simulink model "car"  (R2021a)
settings: Solver=VariableStepAuto  StartTime=0.0  StopTime=10.0  RelTol=1e-3
settings Model: Creator=smrh1  LastModifiedBy=smrh1

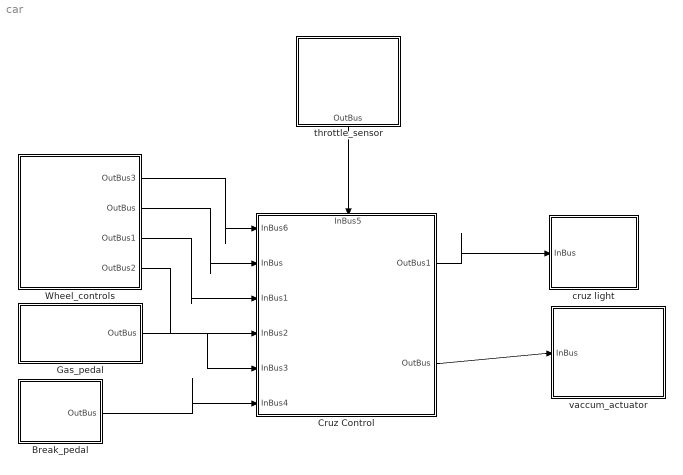
== system car ==
  Break_pedal : Subsystem
      settings: PortSchema="{\"entries\":[{\"content\":{\"headerSize\":26,\"margin\":15,\"minimumSpacing\":25,\"sides\":[{\"content\":{\"connectorIds\":[]},\"type\":\"ConnectorPlacement.EquallySpacedRectSide\",\"uuid\":\"6472313b-455b-4d2f-9eaa-19f0e43a9d41\"},{\"content\":{\"connectorIds\":[\"Out1\"],\"side\":\"RIGHT\"},\"type\":\"ConnectorPlacement.EquallySpacedRectSide\",\"uuid\":\"0bb4b84f-a849-43c7-b807-c30cbc689ce2\"},{\"content\":{\"connectorIds\":[],\"side\":\"TOP\"},\"type\":\"ConnectorPlacement.EquallySpacedRectSide\",\"uuid\":\"136300d7-46ce-438e-aee5-bc57502263b3\"}]},\"type\":\"ConnectorPlacement.EquallySpacedConnector\",\"uuid\":\"08cdd62d-e07b-40ae-9685-722663ceea2d\"}],\"packageUris\":[\"http://schema.mathworks.com/mf0/Connector/R2020b\"],\"version\":\"1.0\"}"
  Cruz Control : Subsystem
      settings: PortSchema="{\"entries\":[{\"content\":{\"headerSize\":26,\"margin\":15,\"minimumSpacing\":25,\"sides\":[{\"content\":{\"connectorIds\":[\"In1\",\"In5\",\"In3\",\"In4\",\"In6\",\"In7\"]},\"type\":\"ConnectorPlacement.EquallySpacedRectSide\",\"uuid\":\"6472313b-455b-4d2f-9eaa-19f0e43a9d41\"},{\"content\":{\"connectorIds\":[\"Out1\",\"Out2\"],\"side\":\"RIGHT\"},\"type\":\"ConnectorPlacement.EquallySpacedRectSide\",\"uuid\":\"0bb4b84f-a849-43c7-b807-c30cbc689ce2\"},{\"content\":{\"connectorIds\":[\"In2\"],\"side\":\"TOP\"},\"type\":\"ConnectorPlacement.EquallySpacedRectSide\",\"uuid\":\"136300d7-46ce-438e-aee5-bc57502263b3\"},{\"content\":{\"connectorIds\":[],\"side\":\"BOTTOM\"},\"type\":\"ConnectorPlacement.EquallySpacedRectSide\",\"uuid\":\"9109190a-ab23-468c-b16c-34fb84e28b1e\"}]},\"type\":\"ConnectorPlacement.EquallySpacedConnector\",\"uuid\":\"08cdd62d-e07b-40ae-9685-722663ceea2d\"}],\"packageUris\":[\"http://schema.mathworks.com/mf0/Connector/R2020b\"],\"version\":\"1.0\"}"
  Gas_pedal : Subsystem
      settings: PortSchema="{\"entries\":[{\"content\":{\"headerSize\":26,\"margin\":15,\"minimumSpacing\":25,\"sides\":[{\"content\":{\"connectorIds\":[]},\"type\":\"ConnectorPlacement.EquallySpacedRectSide\",\"uuid\":\"6472313b-455b-4d2f-9eaa-19f0e43a9d41\"},{\"content\":{\"connectorIds\":[\"Out1\"],\"side\":\"RIGHT\"},\"type\":\"ConnectorPlacement.EquallySpacedRectSide\",\"uuid\":\"0bb4b84f-a849-43c7-b807-c30cbc689ce2\"},{\"content\":{\"connectorIds\":[],\"side\":\"TOP\"},\"type\":\"ConnectorPlacement.EquallySpacedRectSide\",\"uuid\":\"136300d7-46ce-438e-aee5-bc57502263b3\"}]},\"type\":\"ConnectorPlacement.EquallySpacedConnector\",\"uuid\":\"08cdd62d-e07b-40ae-9685-722663ceea2d\"}],\"packageUris\":[\"http://schema.mathworks.com/mf0/Connector/R2020b\"],\"version\":\"1.0\"}"
  Wheel_controls : Subsystem
      settings: PortSchema="{\"entries\":[{\"content\":{\"headerSize\":26,\"margin\":15,\"minimumSpacing\":25,\"sides\":[{\"content\":{\"connectorIds\":[]},\"type\":\"ConnectorPlacement.EquallySpacedRectSide\",\"uuid\":\"af031d74-65d2-4252-81e5-6d9a1fd8149f\"},{\"content\":{\"connectorIds\":[\"Out1\",\"Out2\",\"Out3\",\"Out4\"],\"side\":\"RIGHT\"},\"type\":\"ConnectorPlacement.EquallySpacedRectSide\",\"uuid\":\"daede40a-d3c3-4ef5-9610-a569ab521095\"},{\"content\":{\"connectorIds\":[],\"side\":\"TOP\"},\"type\":\"ConnectorPlacement.EquallySpacedRectSide\",\"uuid\":\"d81e0d84-460b-4569-b916-0cc5afe47905\"}]},\"type\":\"ConnectorPlacement.EquallySpacedConnector\",\"uuid\":\"ddc853b2-7e74-44f1-90da-04896d4738c6\"}],\"packageUris\":[\"http://schema.mathworks.com/mf0/Connector/R2020b\"],\"version\":\"1.0\"}"
  cruz light : Subsystem
      settings: PortSchema="{\"entries\":[{\"content\":{\"headerSize\":26,\"margin\":15,\"minimumSpacing\":25,\"sides\":[{\"content\":{\"connectorIds\":[\"In1\"]},\"type\":\"ConnectorPlacement.EquallySpacedRectSide\",\"uuid\":\"6472313b-455b-4d2f-9eaa-19f0e43a9d41\"},{\"content\":{\"connectorIds\":[],\"side\":\"RIGHT\"},\"type\":\"ConnectorPlacement.EquallySpacedRectSide\",\"uuid\":\"0bb4b84f-a849-43c7-b807-c30cbc689ce2\"},{\"content\":{\"connectorIds\":[],\"side\":\"TOP\"},\"type\":\"ConnectorPlacement.EquallySpacedRectSide\",\"uuid\":\"136300d7-46ce-438e-aee5-bc57502263b3\"}]},\"type\":\"ConnectorPlacement.EquallySpacedConnector\",\"uuid\":\"08cdd62d-e07b-40ae-9685-722663ceea2d\"}],\"packageUris\":[\"http://schema.mathworks.com/mf0/Connector/R2020b\"],\"version\":\"1.0\"}"
  throttle_sensor : Subsystem
      settings: PortSchema="{\"entries\":[{\"content\":{\"headerSize\":26,\"margin\":15,\"minimumSpacing\":25,\"sides\":[{\"content\":{\"connectorIds\":[]},\"type\":\"ConnectorPlacement.EquallySpacedRectSide\",\"uuid\":\"6472313b-455b-4d2f-9eaa-19f0e43a9d41\"},{\"content\":{\"connectorIds\":[],\"side\":\"RIGHT\"},\"type\":\"ConnectorPlacement.EquallySpacedRectSide\",\"uuid\":\"0bb4b84f-a849-43c7-b807-c30cbc689ce2\"},{\"content\":{\"connectorIds\":[],\"side\":\"TOP\"},\"type\":\"ConnectorPlacement.EquallySpacedRectSide\",\"uuid\":\"136300d7-46ce-438e-aee5-bc57502263b3\"},{\"content\":{\"connectorIds\":[\"Out1\"],\"side\":\"BOTTOM\"},\"type\":\"ConnectorPlacement.EquallySpacedRectSide\",\"uuid\":\"8eadb317-004d-496f-aa52-9a68b828bcdc\"}]},\"type\":\"ConnectorPlacement.EquallySpacedConnector\",\"uuid\":\"08cdd62d-e07b-40ae-9685-722663ceea2d\"}],\"packageUris\":[\"http://schema.mathworks.com/mf0/Connector/R2020b\"],\"version\":\"1.0\"}"
  vaccum_actuator : Subsystem
      settings: PortSchema="{\"entries\":[{\"content\":{\"headerSize\":26,\"margin\":15,\"minimumSpacing\":25,\"sides\":[{\"content\":{\"connectorIds\":[\"In1\"]},\"type\":\"ConnectorPlacement.EquallySpacedRectSide\",\"uuid\":\"6472313b-455b-4d2f-9eaa-19f0e43a9d41\"},{\"content\":{\"connectorIds\":[],\"side\":\"RIGHT\"},\"type\":\"ConnectorPlacement.EquallySpacedRectSide\",\"uuid\":\"0bb4b84f-a849-43c7-b807-c30cbc689ce2\"},{\"content\":{\"connectorIds\":[],\"side\":\"TOP\"},\"type\":\"ConnectorPlacement.EquallySpacedRectSide\",\"uuid\":\"136300d7-46ce-438e-aee5-bc57502263b3\"}]},\"type\":\"ConnectorPlacement.EquallySpacedConnector\",\"uuid\":\"08cdd62d-e07b-40ae-9685-722663ceea2d\"}],\"packageUris\":[\"http://schema.mathworks.com/mf0/Connector/R2020b\"],\"version\":\"1.0\"}"
  wires:
  Gas_pedal/1(OutBus) -> Cruz Control/6(InBus3)
  Cruz Control/1(OutBus1) -> cruz light/1(InBus)
  Break_pedal/1(OutBus) -> Cruz Control/7(InBus4)
  Cruz Control/2(OutBus) -> vaccum_actuator/1(InBus)
  throttle_sensor/1(OutBus) -> Cruz Control/2(InBus5)
  Wheel_controls/2(OutBus) -> Cruz Control/5(InBus)
  Wheel_controls/3(OutBus1) -> Cruz Control/3(InBus1)
  Wheel_controls/4(OutBus2) -> Cruz Control/4(InBus2)
  Wheel_controls/1(OutBus3) -> Cruz Control/1(InBus6)

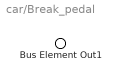
== system car/Break_pedal ==
  Bus Element Out1 : Outport  PortName=OutBus

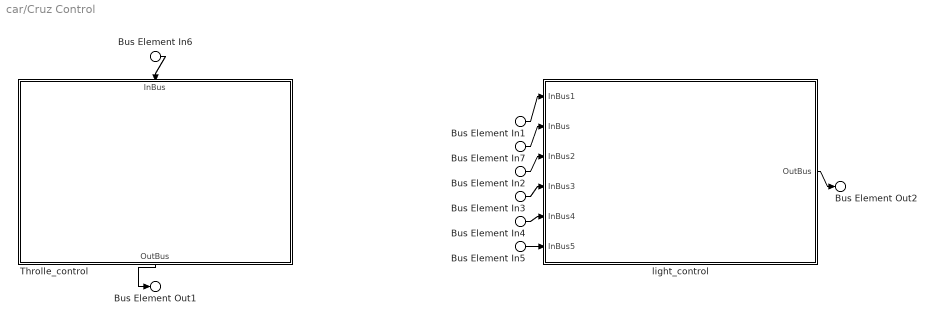
== system car/Cruz Control ==
  Bus Element In7 : Inport  PortName=InBus6
  Bus Element In6 : Inport  Port=2  PortName=InBus5
  Bus Element In2 : Inport  Port=3  PortName=InBus1
  Bus Element In3 : Inport  Port=4  PortName=InBus2
  Bus Element In1 : Inport  Port=5  PortName=InBus
  Bus Element In4 : Inport  Port=6  PortName=InBus3
  Bus Element In5 : Inport  Port=7  PortName=InBus4
  Throlle_control : Subsystem
      settings: PortSchema="{\"entries\":[{\"content\":{\"headerSize\":26,\"margin\":15,\"minimumSpacing\":25,\"sides\":[{\"content\":{\"connectorIds\":[]},\"type\":\"ConnectorPlacement.EquallySpacedRectSide\",\"uuid\":\"6472313b-455b-4d2f-9eaa-19f0e43a9d41\"},{\"content\":{\"connectorIds\":[],\"side\":\"RIGHT\"},\"type\":\"ConnectorPlacement.EquallySpacedRectSide\",\"uuid\":\"0bb4b84f-a849-43c7-b807-c30cbc689ce2\"},{\"content\":{\"connectorIds\":[\"In1\"],\"side\":\"TOP\"},\"type\":\"ConnectorPlacement.EquallySpacedRectSide\",\"uuid\":\"136300d7-46ce-438e-aee5-bc57502263b3\"},{\"content\":{\"connectorIds\":[\"Out1\"],\"side\":\"BOTTOM\"},\"type\":\"ConnectorPlacement.EquallySpacedRectSide\",\"uuid\":\"47a51370-8899-40a2-9cda-cea4c92ab7c8\"}]},\"type\":\"ConnectorPlacement.EquallySpacedConnector\",\"uuid\":\"08cdd62d-e07b-40ae-9685-722663ceea2d\"}],\"packageUris\":[\"http://schema.mathworks.com/mf0/Connector/R2020b\"],\"version\":\"1.0\"}"
  light_control : Subsystem
      settings: PortSchema="{\"entries\":[{\"content\":{\"headerSize\":26,\"margin\":15,\"minimumSpacing\":25,\"sides\":[{\"content\":{\"connectorIds\":[\"In1\",\"In2\",\"In3\",\"In4\",\"In5\",\"In6\"]},\"type\":\"ConnectorPlacement.EquallySpacedRectSide\",\"uuid\":\"6472313b-455b-4d2f-9eaa-19f0e43a9d41\"},{\"content\":{\"connectorIds\":[\"Out1\"],\"side\":\"RIGHT\"},\"type\":\"ConnectorPlacement.EquallySpacedRectSide\",\"uuid\":\"0bb4b84f-a849-43c7-b807-c30cbc689ce2\"},{\"content\":{\"connectorIds\":[],\"side\":\"TOP\"},\"type\":\"ConnectorPlacement.EquallySpacedRectSide\",\"uuid\":\"136300d7-46ce-438e-aee5-bc57502263b3\"}]},\"type\":\"ConnectorPlacement.EquallySpacedConnector\",\"uuid\":\"08cdd62d-e07b-40ae-9685-722663ceea2d\"}],\"packageUris\":[\"http://schema.mathworks.com/mf0/Connector/R2020b\"],\"version\":\"1.0\"}"
  Bus Element Out2 : Outport  PortName=OutBus1
  Bus Element Out1 : Outport  Port=2  PortName=OutBus
  wires:
  Bus Element In7/1 -> light_control/2(InBus)
  Bus Element In1/1 -> light_control/1(InBus1)
  Bus Element In2/1 -> light_control/3(InBus2)
  Bus Element In3/1 -> light_control/4(InBus3)
  Bus Element In4/1 -> light_control/5(InBus4)
  Bus Element In5/1 -> light_control/6(InBus5)
  light_control/1(OutBus) -> Bus Element Out2/1
  Bus Element In6/1 -> Throlle_control/1(InBus)
  Throlle_control/1(OutBus) -> Bus Element Out1/1

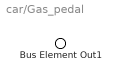
== system car/Gas_pedal ==
  Bus Element Out1 : Outport  PortName=OutBus

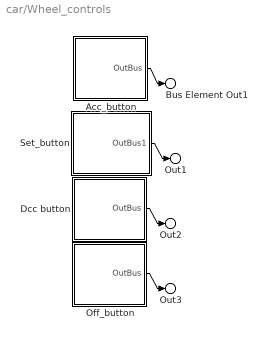
== system car/Wheel_controls ==
  Acc_button : Subsystem
      settings: PortSchema="{\"entries\":[{\"content\":{\"headerSize\":26,\"margin\":15,\"minimumSpacing\":25,\"sides\":[{\"content\":{\"connectorIds\":[]},\"type\":\"ConnectorPlacement.EquallySpacedRectSide\",\"uuid\":\"6472313b-455b-4d2f-9eaa-19f0e43a9d41\"},{\"content\":{\"connectorIds\":[\"Out1\"],\"side\":\"RIGHT\"},\"type\":\"ConnectorPlacement.EquallySpacedRectSide\",\"uuid\":\"0bb4b84f-a849-43c7-b807-c30cbc689ce2\"},{\"content\":{\"connectorIds\":[],\"side\":\"TOP\"},\"type\":\"ConnectorPlacement.EquallySpacedRectSide\",\"uuid\":\"136300d7-46ce-438e-aee5-bc57502263b3\"}]},\"type\":\"ConnectorPlacement.EquallySpacedConnector\",\"uuid\":\"08cdd62d-e07b-40ae-9685-722663ceea2d\"}],\"packageUris\":[\"http://schema.mathworks.com/mf0/Connector/R2020b\"],\"version\":\"1.0\"}"
  Dcc button : Subsystem
      settings: PortSchema="{\"entries\":[{\"content\":{\"headerSize\":26,\"margin\":15,\"minimumSpacing\":25,\"sides\":[{\"content\":{\"connectorIds\":[]},\"type\":\"ConnectorPlacement.EquallySpacedRectSide\",\"uuid\":\"6472313b-455b-4d2f-9eaa-19f0e43a9d41\"},{\"content\":{\"connectorIds\":[\"Out1\"],\"side\":\"RIGHT\"},\"type\":\"ConnectorPlacement.EquallySpacedRectSide\",\"uuid\":\"0bb4b84f-a849-43c7-b807-c30cbc689ce2\"},{\"content\":{\"connectorIds\":[],\"side\":\"TOP\"},\"type\":\"ConnectorPlacement.EquallySpacedRectSide\",\"uuid\":\"136300d7-46ce-438e-aee5-bc57502263b3\"}]},\"type\":\"ConnectorPlacement.EquallySpacedConnector\",\"uuid\":\"08cdd62d-e07b-40ae-9685-722663ceea2d\"}],\"packageUris\":[\"http://schema.mathworks.com/mf0/Connector/R2020b\"],\"version\":\"1.0\"}"
  Off_button : Subsystem
      settings: PortSchema="{\"entries\":[{\"content\":{\"headerSize\":26,\"margin\":15,\"minimumSpacing\":25,\"sides\":[{\"content\":{\"connectorIds\":[]},\"type\":\"ConnectorPlacement.EquallySpacedRectSide\",\"uuid\":\"6472313b-455b-4d2f-9eaa-19f0e43a9d41\"},{\"content\":{\"connectorIds\":[\"Out1\"],\"side\":\"RIGHT\"},\"type\":\"ConnectorPlacement.EquallySpacedRectSide\",\"uuid\":\"0bb4b84f-a849-43c7-b807-c30cbc689ce2\"},{\"content\":{\"connectorIds\":[],\"side\":\"TOP\"},\"type\":\"ConnectorPlacement.EquallySpacedRectSide\",\"uuid\":\"136300d7-46ce-438e-aee5-bc57502263b3\"}]},\"type\":\"ConnectorPlacement.EquallySpacedConnector\",\"uuid\":\"08cdd62d-e07b-40ae-9685-722663ceea2d\"}],\"packageUris\":[\"http://schema.mathworks.com/mf0/Connector/R2020b\"],\"version\":\"1.0\"}"
  Set_button : Subsystem
      settings: PortSchema="{\"entries\":[{\"content\":{\"headerSize\":26,\"margin\":15,\"minimumSpacing\":25,\"sides\":[{\"content\":{\"connectorIds\":[]},\"type\":\"ConnectorPlacement.EquallySpacedRectSide\",\"uuid\":\"6472313b-455b-4d2f-9eaa-19f0e43a9d41\"},{\"content\":{\"connectorIds\":[\"Out1\"],\"side\":\"RIGHT\"},\"type\":\"ConnectorPlacement.EquallySpacedRectSide\",\"uuid\":\"0bb4b84f-a849-43c7-b807-c30cbc689ce2\"},{\"content\":{\"connectorIds\":[],\"side\":\"TOP\"},\"type\":\"ConnectorPlacement.EquallySpacedRectSide\",\"uuid\":\"136300d7-46ce-438e-aee5-bc57502263b3\"},{\"content\":{\"connectorIds\":[],\"side\":\"BOTTOM\"},\"type\":\"ConnectorPlacement.EquallySpacedRectSide\",\"uuid\":\"e062b7e7-d81a-492f-896d-50e5d180cabb\"}]},\"type\":\"ConnectorPlacement.EquallySpacedConnector\",\"uuid\":\"08cdd62d-e07b-40ae-9685-722663ceea2d\"}],\"packageUris\":[\"http://schema.mathworks.com/mf0/Connector/R2020b\"],\"version\":\"1.0\"}"
  Bus Element Out1 : Outport  PortName=OutBus3
  Out1 : Outport  Port=2  PortName=OutBus
  Out2 : Outport  Port=3  PortName=OutBus1
  Out3 : Outport  Port=4  PortName=OutBus2
  wires:
  Set_button/1(OutBus1) -> Out1/1
  Dcc button/1(OutBus) -> Out2/1
  Off_button/1(OutBus) -> Out3/1
  Acc_button/1(OutBus) -> Bus Element Out1/1

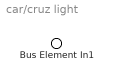
== system car/cruz light ==
  Bus Element In1 : Inport  PortName=InBus

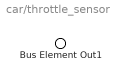
== system car/throttle_sensor ==
  Bus Element Out1 : Outport  PortName=OutBus

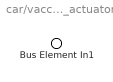
== system car/vaccum_actuator ==
  Bus Element In1 : Inport  PortName=InBus

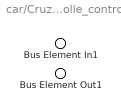
== system car/Cruz Control/Throlle_control ==
  Bus Element In1 : Inport  PortName=InBus
  Bus Element Out1 : Outport  PortName=OutBus

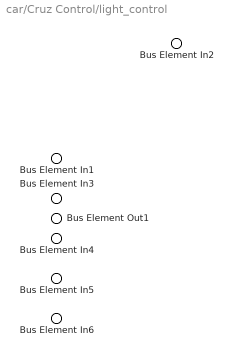
== system car/Cruz Control/light_control ==
  Bus Element In2 : Inport  PortName=InBus1
  Bus Element In1 : Inport  Port=2  PortName=InBus
  Bus Element In3 : Inport  Port=3  PortName=InBus2
  Bus Element In4 : Inport  Port=4  PortName=InBus3
  Bus Element In5 : Inport  Port=5  PortName=InBus4
  Bus Element In6 : Inport  Port=6  PortName=InBus5
  Bus Element Out1 : Outport  PortName=OutBus

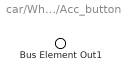
== system car/Wheel_controls/Acc_button ==
  Bus Element Out1 : Outport  PortName=OutBus

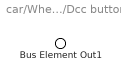
== system car/Wheel_controls/Dcc button ==
  Bus Element Out1 : Outport  PortName=OutBus

== system car/Wheel_controls/Off_button ==
  Bus Element Out1 : Outport  PortName=OutBus

== system car/Wheel_controls/Set_button ==
  Bus Element Out2 : Outport  PortName=OutBus1
